simulink model "Lab7_Ex2_Template_gr2159"  (R2020a)
settings: Solver=ode1  StartTime=0.0  StopTime=60  FixedStep=0.002  RelTol=1e-3  EnableMultiTasking=on
libraries: quarc_library x4
settings Model: ExtModeTrigDuration=10000  Creator=merii  LastModifiedBy=Admin
settings SolverCC: PositivePriorityOrder=on
settings DataIOCC: ReturnWorkspaceOutputs=off
settings OptimizationCC: LifeSpan=inf
settings DebuggingCC: ArithmeticOperatorsInVariantConditions=warning
settings SFSimCC: SimUseLocalCustomCode=off  CustomCodeUndefinedFunction=UseInterfaceOnly
settings RTWCC: Description=QUARC Win64 Target  SystemTargetFile=quarc_win64.tlc  TemplateMakefile=quarc_default_tmf  RTWUseLocalCustomCode=off
settings CodeAppCC: StateflowObjectComments=on
settings STFCustomTargetCC: TargetPreCompLibLocation=C:\PROGRA~3\QUARC\lib\2020a\win64\release  TargetLangStandard=C99 (ISO)  ConcurrentExecutionCompliant=on  GRTInterface=on  SystemTargetFile=quarc_win64.tlc
settings GRTTargetCC: TargetPreCompLibLocation=C:\PROGRA~3\QUARC\lib\2020a\win64\release  ParMdlRefBuildCompliant=off  CompOptLevelCompliant=off  CombineOutputUpdateFcns=off  MatFileLogging=off  CPPClassGenCompliant=off  GRTInterface=on  UseToolchainInfoCompliant=off  ExtMode=on  ExtModeMexFile=quarc_comm
settings ConfigComp: CovMetricSettings=dswe

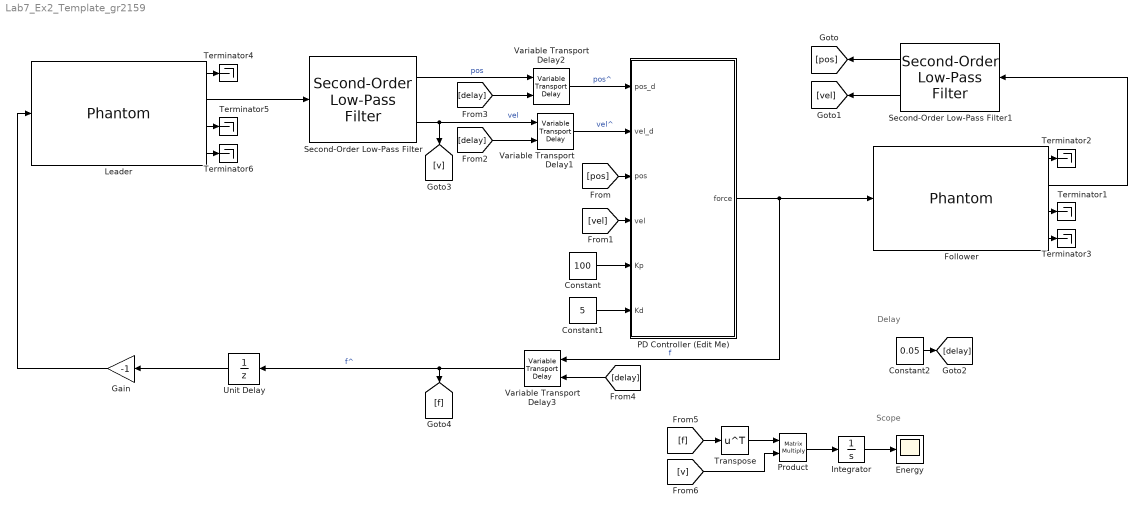
== system Lab7_Ex2_Template_gr2159 ==
  note: Scope
  note: Delay
  Constant : Constant  Value=100
  Constant1 : Constant  Value=5
  Constant2 : Constant  Value=0.05
  Energy : Scope
  Follower : quarc_library/Devices/Third-Party/SensAble/Phantom/Phantom  device_name=Right Device  output_type=Positions and Gimbal Angles  input_type=Cartesian space  velocity_limit_option=on  velocity_limit=1200  is_7dof=off  sample_time=-1
      settings: AttributesFormatString=(%<device_name>)  SourceProductName=QUARC Targets
  Gain : Gain  Gain=-1
  Integrator : Integrator
  Leader : quarc_library/Devices/Third-Party/SensAble/Phantom/Phantom  device_name=Left Device  output_type=Positions and Gimbal Angles  input_type=Cartesian space  velocity_limit_option=on  velocity_limit=1200  is_7dof=off  sample_time=-1
      settings: AttributesFormatString=(%<device_name>)  SourceProductName=QUARC Targets
  PD Controller (Edit Me) : MATLAB Function  TreatAsAtomicUnit=on
  Product : Product  Multiplication=Matrix(*)
  Second-Order Low-Pass Filter : quarc_library/Continuous/Second-Order Low-Pass Filter  params_source=Internal (dialog parameters)  input_width=50  input_zeta=1  input_init=0
  Second-Order Low-Pass Filter1 : quarc_library/Continuous/Second-Order Low-Pass Filter  params_source=Internal (dialog parameters)  input_width=50  input_zeta=1  input_init=0
  Terminator{1..6} (6 alike) : Terminator
  Transpose : Math  Operator=transpose  SaturateOnIntegerOverflow=on
  Unit Delay : UnitDelay  SampleTime=-1  HasFrameUpgradeWarning=on
  Variable Transport Delay1 : VariableTransportDelay  MaximumDelay=10  ZeroDelay=on
  Variable Transport Delay2 : VariableTransportDelay  MaximumDelay=10  ZeroDelay=on
  Variable Transport Delay3 : VariableTransportDelay  MaximumDelay=10  ZeroDelay=on
  wires:
  Leader/2 -> Second-Order Low-Pass Filter/1
  Second-Order Low-Pass Filter/1 -> Variable Transport Delay2/1  "pos"
  Second-Order Low-Pass Filter/2 -> [v], Variable Transport Delay1/1  "vel"
  PD Controller (Edit Me)/1(force) -> Follower/1, Variable Transport Delay3/1  "f"
  Follower/2 -> Second-Order Low-Pass Filter1/1
  Second-Order Low-Pass Filter1/1 -> [pos]
  Second-Order Low-Pass Filter1/2 -> [vel]
  [pos] -> PD Controller (Edit Me)/3(pos)
  [vel] -> PD Controller (Edit Me)/4(vel)
  Constant/1 -> PD Controller (Edit Me)/5(Kp)
  Constant1/1 -> PD Controller (Edit Me)/6(Kd)
  Unit Delay/1 -> Gain/1
  Gain/1 -> Leader/1
  [delay] -> Variable Transport Delay1/2
  Variable Transport Delay1/1 -> PD Controller (Edit Me)/2(vel_d)  "vel^"
  [delay] -> Variable Transport Delay2/2
  Variable Transport Delay2/1 -> PD Controller (Edit Me)/1(pos_d)  "pos^"
  [delay] -> Variable Transport Delay3/2
  Variable Transport Delay3/1 -> [f], Unit Delay/1  "f^"
  Constant2/1 -> [delay]
  Follower/1 -> Terminator2/1
  Follower/3 -> Terminator1/1
  Follower/4 -> Terminator3/1
  Leader/1 -> Terminator4/1
  Leader/3 -> Terminator5/1
  Leader/4 -> Terminator6/1
  [f] -> Transpose/1
  Transpose/1 -> Product/1
  [v] -> Product/2
  Product/1 -> Integrator/1
  Integrator/1 -> Energy/1

== matlab function Lab7_Ex2_Template_gr2159/PD Controller (Edit Me) ==
  data: pos_d input; force output; vel_d input; pos input; vel input; Kp input; Kd input
function force = fcn(pos_d, vel_d, pos, vel, Kp, Kd)

%Create PD Controller

force=Kp*(pos_d-pos)+Kd*(vel_d-vel);

end
